simulink model "DriverInLoopSpeedgoat"  (R2021a)
settings: Solver=ode3  StartTime=0.0  StopTime=30  FixedStep=1e-3  RelTol=5e-3  EnableMultiTasking=on
StartFcn:
  | % tic
  | % tg2.start;
StopFcn:
  | % tg2.stop;
  | % toc
model workspace (MAT data in the model file):
  A_mu = 10
  B_reff = 8.386
  Cz = 7766.25
  DCT_Param : object (value not decoded)
  DLC_XEnd = 236.9
  DLC_XStart = 175.9
  DLC_YStart = 3.2153
  D_reff = 0.25826
  Downshift_Speeds = [9.5625 12.9375 16.3125 19.6875 23.0625 26.4375 29.8125 33.1875 36.5625 39.9375 43.3125 46.6875 ... (16 elements, 4x4)]
  EngRevLim = 7000
  Pedal_Positions = [0.1 0.4 0.5 0.9]
  SUS : object (value not decoded)
  Upshift_Speeds = [12.9375 16.3125 19.6875 33 26.4375 29.8125 33.1875 52.5 39.9375 43.3125 46.6875 77.25 ... (16 elements, 4x4)]
  VEH : object (value not decoded)
  V_o = 16.7
  V_xlow = 1
  WH : object (value not decoded)
  a = 1.4
  alpha_max = 1.5
  alpha_min = -1.5
  b = 1.8
  c_zo = 209651
  epsilon = 0.1
  h = 0.134
  path : object (value not decoded)
  pio = 220000
  q_Fcx = 0
  q_Fz2 = 15.4
  q_Fzy = 0
  q_reo = 0.9974
  q_sx1 = -0.007764
  q_sx10 = 0.2824
  q_sx11 = 5.349
  q_sx12 = 0
  q_sx13 = 0
  q_sx14 = 0
  q_sx2 = 1.1915
  q_sx3 = 0.013948
  q_sx4 = 4.912
  q_sx5 = 1.02
  q_sx6 = 22.83
  q_sx7 = 0.7104
  q_sx8 = -0.023393
  q_sx9 = 0.6581
  q_sy1 = 0.00702
  q_sy2 = 0
  q_sy3 = 0.001515
  q_sy4 = 8.514e-05
  q_sy5 = 0
  q_sy6 = 0
  q_sy7 = 0.9008
  q_sy8 = -0.4089
  q_v1 = 0.0007742
  q_v2 = 0.04667
  r_Bx1 = 12.531
  r_Bx2 = 9.532
  r_Bx3 = 0
  r_By1 = 10.615
  r_By2 = 7.705
  r_By3 = 3.433e-06
  r_By4 = 0
  r_Cx1 = 1.019
  r_Cy1 = 1.0585
  r_Ex1 = -0.4487
  r_Ex2 = -0.4726
  r_Ey1 = 0.3132
  r_Ey2 = 7.63e-06
  r_Hx1 = 0.0002374
  r_Hy1 = 0.011646
  r_Hy2 = 7.63e-06
  r_Vy1 = 0.05654
  r_Vy2 = 7.63e-06
  r_Vy3 = 0
  r_Vy4 = 99.9
  r_Vy5 = 2
  r_Vy6 = 15.814
  r_o = 0.3135
  vehWidth = 2
  w = 1
  xdot_ref = 13.4112
values from neighbouring files (symbols this model uses):
  stop_pedal = 20    [config_test.m]
symbols that are objects in the model workspace (value not decoded): VEH
undefined symbols (not defined in the file or in its folder): ESP_mode
libraries: autolibutils x7, simulink x6, slrealtimeutilitieslib x2, slrealtimeiplib x2, sim3dlib x1, sim3dautolib x1, pid_lib x1, slrealtimeobsoletelib x1, dspstat3 x1
(part 2 of 2)

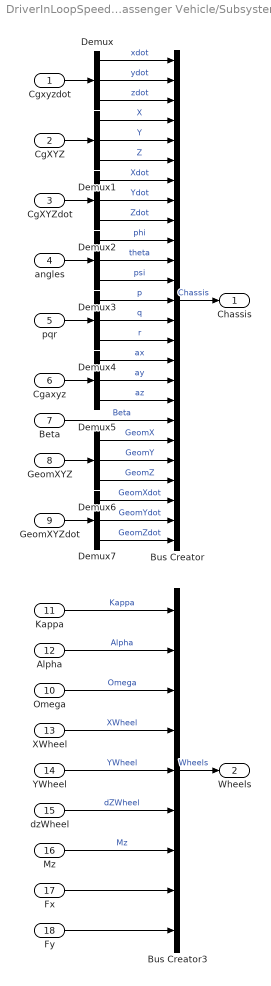
== system DriverInLoopSpeedgoat/Passenger Vehicle/Subsystem4 ==
  Cgxyzdot : Inport
  CgXYZ : Inport  Port=2
  CgXYZdot : Inport  Port=3
  angles : Inport  Port=4
  pqr : Inport  Port=5
  Cgaxyz : Inport  Port=6
  Beta : Inport  Port=7
  GeomXYZ : Inport  Port=8
  GeomXYZdot : Inport  Port=9
  Omega : Inport  Port=10
  Kappa : Inport  Port=11
  Alpha : Inport  Port=12
  XWheel : Inport  Port=13
  YWheel : Inport  Port=14
  dzWheel : Inport  Port=15
  Mz : Inport  Port=16
  Fx : Inport  Port=17
  Fy : Inport  Port=18
  Bus Creator : BusCreator  Inputs=25
  Bus Creator3 : BusCreator  Inputs=9
  Demux{,1..7} (8 alike) : Demux  Outputs=3
  Chassis : Outport  VectorParamsAs1DForOutWhenUnconnected=off
  Wheels : Outport  Port=2  VectorParamsAs1DForOutWhenUnconnected=off
  wires:
  Bus Creator/1 -> Chassis/1  "Chassis"
  Omega/1 -> Bus Creator3/3  "Omega"
  dzWheel/1 -> Bus Creator3/6  "dZWheel"
  Kappa/1 -> Bus Creator3/1  "Kappa"
  Bus Creator3/1 -> Wheels/1  "Wheels"
  YWheel/1 -> Bus Creator3/5  "YWheel"
  XWheel/1 -> Bus Creator3/4  "XWheel"
  Alpha/1 -> Bus Creator3/2  "Alpha"
  Cgxyzdot/1 -> Demux/1
  CgXYZ/1 -> Demux1/1
  CgXYZdot/1 -> Demux2/1
  angles/1 -> Demux3/1
  pqr/1 -> Demux4/1
  Cgaxyz/1 -> Demux5/1
  GeomXYZdot/1 -> Demux7/1
  GeomXYZ/1 -> Demux6/1
  Demux/1 -> Bus Creator/1  "xdot"
  Demux/2 -> Bus Creator/2  "ydot"
  Demux/3 -> Bus Creator/3  "zdot"
  Demux1/1 -> Bus Creator/4  "X"
  Demux1/2 -> Bus Creator/5  "Y"
  Demux1/3 -> Bus Creator/6  "Z"
  Demux2/1 -> Bus Creator/7  "Xdot"
  Demux2/2 -> Bus Creator/8  "Ydot"
  Demux2/3 -> Bus Creator/9  "Zdot"
  Demux3/1 -> Bus Creator/10  "phi"
  Demux3/2 -> Bus Creator/11  "theta"
  Demux3/3 -> Bus Creator/12  "psi"
  Demux4/1 -> Bus Creator/13  "p"
  Demux4/2 -> Bus Creator/14  "q"
  Demux4/3 -> Bus Creator/15  "r"
  Demux5/1 -> Bus Creator/16  "ax"
  Demux5/2 -> Bus Creator/17  "ay"
  Demux5/3 -> Bus Creator/18  "az"
  Beta/1 -> Bus Creator/19  "Beta"
  Demux6/1 -> Bus Creator/20  "GeomX"
  Demux6/2 -> Bus Creator/21  "GeomY"
  Demux6/3 -> Bus Creator/22  "GeomZ"
  Demux7/1 -> Bus Creator/23  "GeomXdot"
  Demux7/2 -> Bus Creator/24  "GeomYdot"
  Demux7/3 -> Bus Creator/25  "GeomZdot"
  Mz/1 -> Bus Creator3/7  "Mz"
  Fx/1 -> Bus Creator3/8
  Fy/1 -> Bus Creator3/9

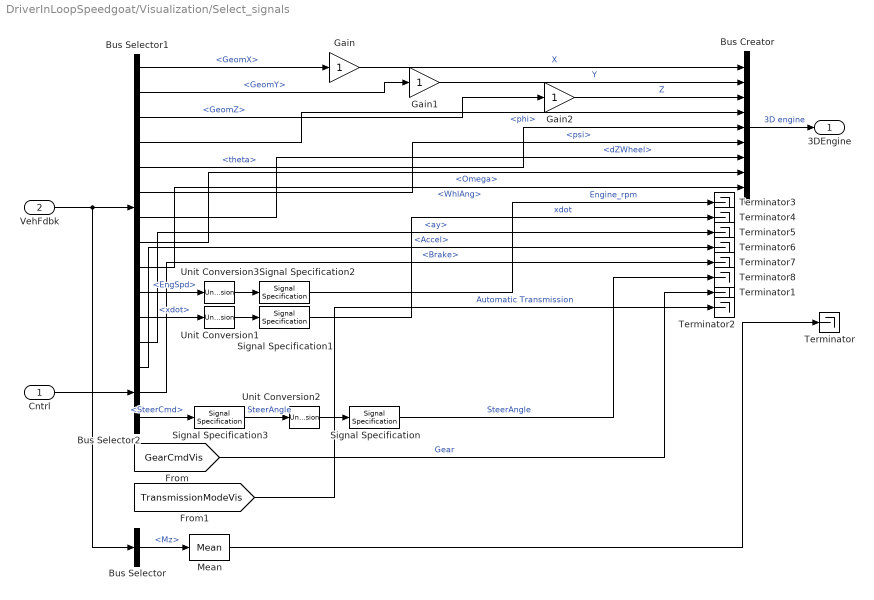
== system DriverInLoopSpeedgoat/Visualization/Select_signals ==
  Cntrl : Inport
  VehFdbk : Inport  Port=2
  Bus Creator : BusCreator  Inputs=9
  Bus Selector : BusSelector  OutputSignals=Wheels.Mz
  Bus Selector1 : BusSelector  OutputSignals=Body.GeomX,Body.GeomY,Body.GeomZ,Body.phi,Body.theta,Body.psi,Wheels.dZWheel,Wheels.Omega,Driveline.WhlAng,Driveline.EngSpd,Body.xdot,Body.ay
  Bus Selector2 : BusSelector  OutputSignals=Accel,Brake,SteerCmd
  Gain : Gain
  Gain1 : Gain
  Gain2 : Gain
  Mean : dspstat3/Mean  run=off  InputProcessing=Columns as channels (frame based)  reset_popup=None  directionMode=Each column  dimension=1  roiEnable=off  roiType=Rectangles  roiPortion=Entire ROI  roiOutput=Individual statistics for each ROI  roiFlag=off  roundingMode=Floor  overflowMode=off  outputDataTypeStr=Inherit: Same as accumulator  outputMin=[]  outputMax=[]  outputLastDataTypeStr=Inherit: Same as accumulator
  Signal Specification : SignalSpecification  Unit=deg
  Signal Specification1 : SignalSpecification  Unit=mph
  Signal Specification2 : SignalSpecification  Unit=rpm
  Signal Specification3 : SignalSpecification  Unit=deg
  Terminator{,1..8} (9 alike) : Terminator
  Unit Conversion1 : UnitConversion
  Unit Conversion2 : UnitConversion
  Unit Conversion3 : UnitConversion
  3DEngine : Outport
  wires:
  Bus Selector1/11 -> Unit Conversion1/1  "<xdot>"
  Signal Specification2/1 -> Terminator3/1  "Engine_rpm"
  Unit Conversion3/1 -> Signal Specification2/1
  Bus Selector2/1 -> Terminator6/1  "<Accel>"
  Bus Selector1/12 -> Terminator5/1  "<ay>"
  VehFdbk/1 -> Bus Selector1/1, Bus Selector/1
  Unit Conversion2/1 -> Signal Specification/1
  Signal Specification/1 -> Terminator8/1  "SteerAngle"
  Bus Selector1/8 -> Bus Creator/8  "<Omega>"
  Bus Selector1/4 -> Bus Creator/4  "<phi>"
  Cntrl/1 -> Bus Selector2/1
  Bus Selector1/10 -> Unit Conversion3/1  "<EngSpd>"
  Unit Conversion1/1 -> Signal Specification1/1
  Bus Selector2/3 -> Signal Specification3/1  "<SteerCmd>"
  Bus Selector1/5 -> Bus Creator/5  "<theta>"
  Bus Selector1/7 -> Bus Creator/7  "<dZWheel>"
  Bus Selector2/2 -> Terminator7/1  "<Brake>"
  Bus Selector1/6 -> Bus Creator/6  "<psi>"
  Bus Selector1/9 -> Bus Creator/9  "<WhlAng>"
  Signal Specification1/1 -> Terminator4/1  "xdot"
  Bus Selector/1 -> Mean/1  "<Mz>"
  Signal Specification3/1 -> Unit Conversion2/1  "SteerAngle"
  Bus Creator/1 -> 3DEngine/1  "3D engine"
  Mean/1 -> Terminator/1
  Bus Selector1/3 -> Gain2/1  "<GeomZ>"
  Bus Selector1/2 -> Gain1/1  "<GeomY>"
  [GearCmdVis] -> Terminator1/1  "Gear"
  Bus Selector1/1 -> Gain/1  "<GeomX>"
  [TransmissionModeVis] -> Terminator2/1  "Automatic Transmission"
  Gain/1 -> Bus Creator/1  "X"
  Gain1/1 -> Bus Creator/2  "Y"
  Gain2/1 -> Bus Creator/3  "Z"

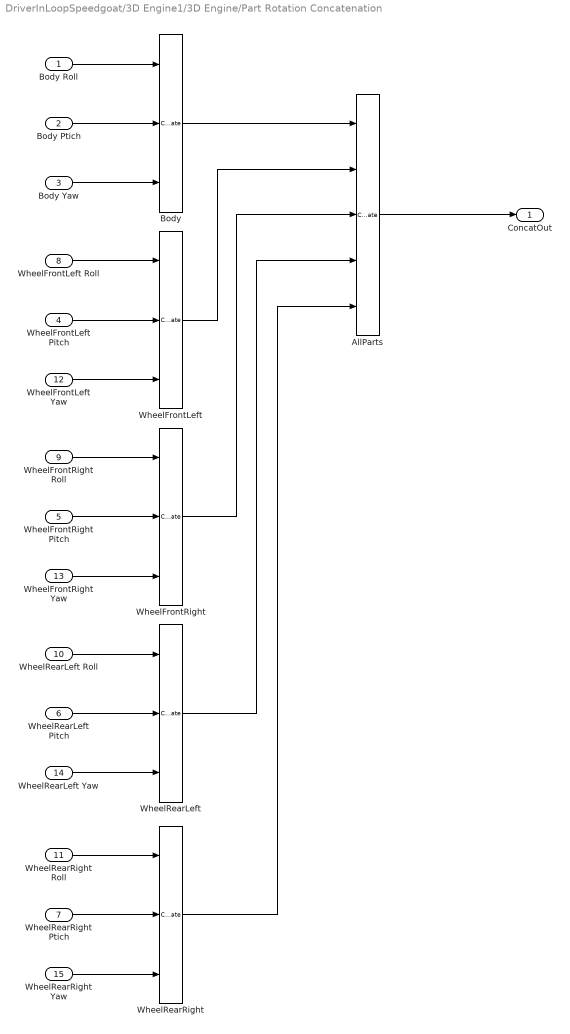
== system DriverInLoopSpeedgoat/3D Engine1/3D Engine/Part Rotation Concatenation ==
  Body Roll : Inport
  Body Ptich : Inport  Port=2
  Body Yaw : Inport  Port=3
  WheelFrontLeft Pitch : Inport  Port=4
  WheelFrontRight Pitch : Inport  Port=5
  WheelRearLeft Pitch : Inport  Port=6
  WheelRearRight Ptich : Inport  Port=7
  WheelFrontLeft Roll : Inport  Port=8
  WheelFrontRight Roll : Inport  Port=9
  WheelRearLeft Roll : Inport  Port=10
  WheelRearRight Roll : Inport  Port=11
  WheelFrontLeft Yaw : Inport  Port=12
  WheelFrontRight Yaw : Inport  Port=13
  WheelRearLeft Yaw : Inport  Port=14
  WheelRearRight Yaw : Inport  Port=15
  AllParts : Concatenate  NumInputs=5  Mode=Multidimensional array
  Body : Concatenate  NumInputs=3  Mode=Multidimensional array  ConcatenateDimension=2
  WheelFrontLeft : Concatenate  NumInputs=3  Mode=Multidimensional array  ConcatenateDimension=2
  WheelFrontRight : Concatenate  NumInputs=3  Mode=Multidimensional array  ConcatenateDimension=2
  WheelRearLeft : Concatenate  NumInputs=3  Mode=Multidimensional array  ConcatenateDimension=2
  WheelRearRight : Concatenate  NumInputs=3  Mode=Multidimensional array  ConcatenateDimension=2
  ConcatOut : Outport  VectorParamsAs1DForOutWhenUnconnected=off
  wires:
  Body Yaw/1 -> Body/3
  WheelFrontLeft Yaw/1 -> WheelFrontLeft/3
  WheelFrontLeft/1 -> AllParts/2
  Body/1 -> AllParts/1
  WheelRearLeft/1 -> AllParts/4
  WheelFrontRight/1 -> AllParts/3
  WheelRearRight Yaw/1 -> WheelRearRight/3
  WheelRearLeft Yaw/1 -> WheelRearLeft/3
  AllParts/1 -> ConcatOut/1
  WheelRearRight/1 -> AllParts/5
  WheelFrontRight Yaw/1 -> WheelFrontRight/3
  Body Roll/1 -> Body/1
  Body Ptich/1 -> Body/2
  WheelFrontLeft Pitch/1 -> WheelFrontLeft/2
  WheelFrontLeft Roll/1 -> WheelFrontLeft/1
  WheelFrontRight Roll/1 -> WheelFrontRight/1
  WheelFrontRight Pitch/1 -> WheelFrontRight/2
  WheelRearLeft Roll/1 -> WheelRearLeft/1
  WheelRearLeft Pitch/1 -> WheelRearLeft/2
  WheelRearRight Roll/1 -> WheelRearRight/1
  WheelRearRight Ptich/1 -> WheelRearRight/2

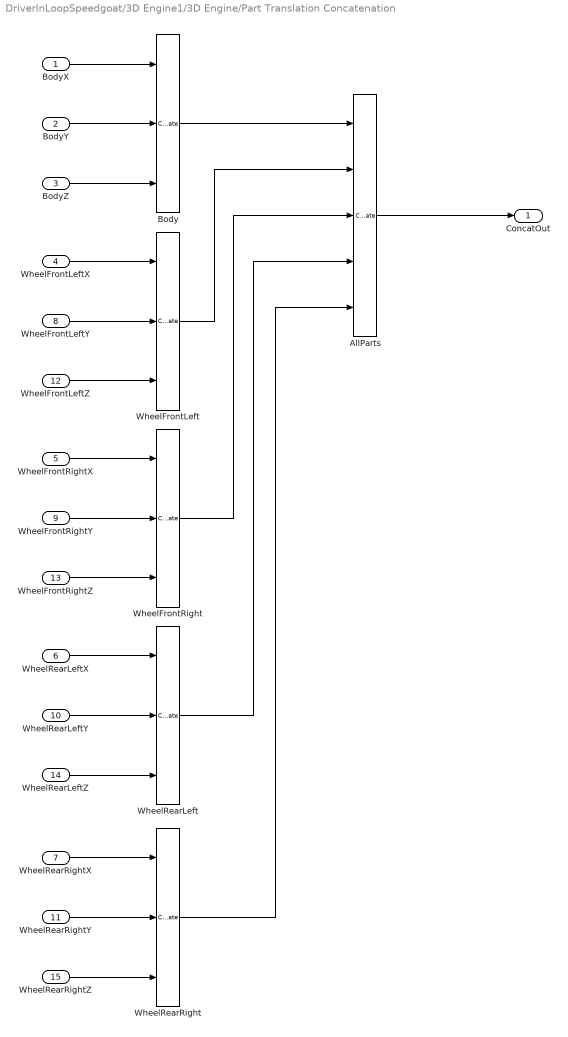
== system DriverInLoopSpeedgoat/3D Engine1/3D Engine/Part Translation Concatenation ==
  BodyX : Inport
  BodyY : Inport  Port=2
  BodyZ : Inport  Port=3
  WheelFrontLeftX : Inport  Port=4
  WheelFrontRightX : Inport  Port=5
  WheelRearLeftX : Inport  Port=6
  WheelRearRightX : Inport  Port=7
  WheelFrontLeftY : Inport  Port=8
  WheelFrontRightY : Inport  Port=9
  WheelRearLeftY : Inport  Port=10
  WheelRearRightY : Inport  Port=11
  WheelFrontLeftZ : Inport  Port=12
  WheelFrontRightZ : Inport  Port=13
  WheelRearLeftZ : Inport  Port=14
  WheelRearRightZ : Inport  Port=15
  AllParts : Concatenate  NumInputs=5  Mode=Multidimensional array
  Body : Concatenate  NumInputs=3  Mode=Multidimensional array  ConcatenateDimension=2
  WheelFrontLeft : Concatenate  NumInputs=3  Mode=Multidimensional array  ConcatenateDimension=2
  WheelFrontRight : Concatenate  NumInputs=3  Mode=Multidimensional array  ConcatenateDimension=2
  WheelRearLeft : Concatenate  NumInputs=3  Mode=Multidimensional array  ConcatenateDimension=2
  WheelRearRight : Concatenate  NumInputs=3  Mode=Multidimensional array  ConcatenateDimension=2
  ConcatOut : Outport  VectorParamsAs1DForOutWhenUnconnected=off
  wires:
  BodyX/1 -> Body/1
  BodyZ/1 -> Body/3
  WheelFrontLeftX/1 -> WheelFrontLeft/1
  WheelFrontLeftZ/1 -> WheelFrontLeft/3
  WheelFrontLeftY/1 -> WheelFrontLeft/2
  BodyY/1 -> Body/2
  WheelFrontLeft/1 -> AllParts/2
  WheelRearRightX/1 -> WheelRearRight/1
  Body/1 -> AllParts/1
  WheelRearLeft/1 -> AllParts/4
  WheelFrontRight/1 -> AllParts/3
  WheelRearRightZ/1 -> WheelRearRight/3
  WheelFrontRightY/1 -> WheelFrontRight/2
  WheelFrontRightX/1 -> WheelFrontRight/1
  WheelRearRightY/1 -> WheelRearRight/2
  WheelRearLeftZ/1 -> WheelRearLeft/3
  AllParts/1 -> ConcatOut/1
  WheelRearLeftY/1 -> WheelRearLeft/2
  WheelRearRight/1 -> AllParts/5
  WheelRearLeftX/1 -> WheelRearLeft/1
  WheelFrontRightZ/1 -> WheelFrontRight/3

== system DriverInLoopSpeedgoat/3D Engine1/3D Engine/Scale ==
  Constant{1..12,17,32..33} (15 alike) : Constant  OutDataTypeStr=single
  PartConcatenation : Subsystem
  ScaleOut : Outport  VectorParamsAs1DForOutWhenUnconnected=off
  wires:
  Constant10/1 -> PartConcatenation/15(WheelRearRightZ)
  Constant9/1 -> PartConcatenation/14(WheelRearRightY)
  Constant11/1 -> PartConcatenation/13(WheelRearRightX)
  Constant7/1 -> PartConcatenation/12(WheelRearLeftZ)
  Constant6/1 -> PartConcatenation/11(WheelRearLeftY)
  Constant8/1 -> PartConcatenation/10(WheelRearLeftX)
  Constant4/1 -> PartConcatenation/9(WheelFrontRightZ)
  Constant3/1 -> PartConcatenation/8(WheelFrontRightY)
  Constant5/1 -> PartConcatenation/7(WheelFrontRightX)
  Constant2/1 -> PartConcatenation/6(WheelFrontLeftZ)
  Constant1/1 -> PartConcatenation/5(WheelFrontLeftY)
  Constant33/1 -> PartConcatenation/4(WheelFrontLeftX)
  Constant32/1 -> PartConcatenation/3(BodyZ)
  Constant17/1 -> PartConcatenation/2(BodyY)
  Constant12/1 -> PartConcatenation/1(BodyX)
  PartConcatenation/1(ConcatOut) -> ScaleOut/1

== system DriverInLoopSpeedgoat/Controllers/Brake Controller/Bang Bang ABS ==
  Pref : Inport
  xdot : Inport  Port=2
  <Kappa> : Inport  Port=3
  Abs : Abs
  Add : Sum  Inputs=-+
  Bang-bang controller : Subsystem  mask(Sign){}
      mask help: y = sign(x)
      mask Help: Sign Function:\n\t\t\ty = 1 if x > 0\n\t\t\ty = 0 if x = 0\n\t\t\ty = -1 if x < 0
      mask Display: plot(-50,-50,50,50,[-50,50],[0,0],[0,0],[-50,50],[-40,0],[-30,-30],[0,40],[30,30])
  Compare To Constant : simulink/Logic and Bit Operations/Compare To Constant  relop=>=  const=.2  OutDataTypeStr=boolean
  Compare To Constant1 : simulink/Logic and Bit Operations/Compare To Constant  relop=>=  const=.75  OutDataTypeStr=boolean
  Compare To Constant2 : simulink/Logic and Bit Operations/Compare To Constant  relop=>=  const=.5  OutDataTypeStr=boolean
  Constant : Constant  Value=.25
  Debounce : autolibutils/Debounce  DbcOn_Cnts=.1*.001  DbcOff_Cnts=.1*.001  aMode=aMode
      settings: SourceProductBaseCode=PW,DR,MT,UV,VE
  Gain : Gain  Gain=200
  Logical Operator : Logic  Inputs=3  AllPortsSameDT=off  OutDataTypeStr=boolean
  Rate Transition : RateTransition  OutPortSampleTime=.001
  Rate Transition1 : RateTransition
  Switch : Switch  Criteria=u2 > Threshold  ZeroCross=off
  PCmd : Outport  VectorParamsAs1DForOutWhenUnconnected=off
  wires:
  Bang-bang controller/1(out_1) -> Gain/1
  Add/1 -> Bang-bang controller/1(in_1)
  Rate Transition1/1 -> PCmd/1
  <Kappa>/1 -> Rate Transition/1
  Pref/1 -> Switch/3, Compare To Constant1/1  "Pref"
  Constant/1 -> Add/2  "slip ref"
  Switch/1 -> Rate Transition1/1
  Rate Transition/1 -> Add/1, Compare To Constant/1
  Logical Operator/1 -> Debounce/1
  Compare To Constant/1 -> Logical Operator/2
  Compare To Constant1/1 -> Logical Operator/3
  Debounce/1 -> Switch/2
  xdot/1 -> Abs/1
  Abs/1 -> Compare To Constant2/1
  Compare To Constant2/1 -> Logical Operator/1
  Gain/1 -> Switch/1

== system DriverInLoopSpeedgoat/Controllers/ECU/Rev Limiter Control ==
  TrqCmd : Inport
  EngSpd : Inport  Port=2
  1-D Lookup Table : Lookup_n-D  NumberOfTableDimensions=1  BreakpointsForDimension1=[1 1.01]  Table=[1 0]  ExtrapMethod=Clip  InternalRulePriority=Speed  RndMeth=Simplest  InputSameDT=on
  Constant : Constant  Value=EngRevLim
  Product : Product
  Product1 : Product  Inputs=*/
  TrqCmdRevLimited : Outport  VectorParamsAs1DForOutWhenUnconnected=off
  wires:
  EngSpd/1 -> Product1/1
  Product/1 -> TrqCmdRevLimited/1
  1-D Lookup Table/1 -> Product/2
  TrqCmd/1 -> Product/1
  Constant/1 -> Product1/2
  Product1/1 -> 1-D Lookup Table/1

== system DriverInLoopSpeedgoat/Controllers/Transmission Controller/Automatic ==
  Accel : Inport
  EngSpd : Inport  Port=2  Unit=rad/s
  PrpSpd : Inport  Port=3
  Action Port : ActionPort  ActionPortLabel=case [ 1 ]:
  Neutral Select : Subsystem
  Prop Shaft Speed LPF : DiscreteTransferFcn  Numerator=[0.000000000000000 0.009950166250832 ]  Denominator=[1.000000000000000 -0.990049833749168 ]  mask(DiscretizedDiscreteTransferFcn){}
      mask init:
      | %zoh
  Signal Specification : SignalSpecification  Unit=rpm
  TCM Shift Controller : Stateflow chart  TreatAsAtomicUnit=on
  Unit Conversion : UnitConversion
  prop speed to vehicle speed : Gain  Gain=0.45
  Gear : Outport  VectorParamsAs1DForOutWhenUnconnected=off
  wires:
  TCM Shift Controller/1(GearCmd) -> Gear/1
  Unit Conversion/1 -> Signal Specification/1
  PrpSpd/1 -> Prop Shaft Speed LPF/1
  Signal Specification/1 -> Neutral Select/2(EngSpd)  "EngSpd"
  EngSpd/1 -> Unit Conversion/1
  Accel/1 -> Neutral Select/1(AccCmd), TCM Shift Controller/2(pedal)  "AccCmd"
  Prop Shaft Speed LPF/1 -> prop speed to vehicle speed/1
  prop speed to vehicle speed/1 -> TCM Shift Controller/1(speed)
  Neutral Select/1(Neutral Select) -> TCM Shift Controller/3(Neutral)

== system DriverInLoopSpeedgoat/Controllers/Transmission Controller/Paddles ==
  UpReq : Inport
  DownReq : Inport  Port=2  Unit=rad/s
  Action Port : ActionPort  ActionPortLabel=case [ 0 ]:
  Add1 : Sum  Inputs=+-+
  Current Gear : UnitDelay  SampleTime=-1  HasFrameUpgradeWarning=on
  Data Type Conversion2 : DataTypeConversion  OutDataTypeStr=int8
  Debounce : autolibutils/Debounce  DbcOn_Cnts=10  DbcOff_Cnts=10  aMode=aMode
      settings: SourceProductBaseCode=PW,DR,MT,UV,VE
  Debounce1 : autolibutils/Debounce  DbcOn_Cnts=10  DbcOff_Cnts=10  aMode=aMode
      settings: SourceProductBaseCode=PW,DR,MT,UV,VE
  Demux : Demux  Outputs=2
  Detect Increase2 : simulink/Logic and Bit Operations/Detect Increase  vinit=0.0  OutDataTypeStr=boolean
  Logical Operator1 : Logic  Operator=XOR  Inputs=1  AllPortsSameDT=off  OutDataTypeStr=boolean
  Mux : Mux  Inputs=2
  Saturation : Saturate  UpperLimit=5  LowerLimit=-1
  Switch2 : Switch  Criteria=u2 > Threshold
  Gear : Outport  VectorParamsAs1DForOutWhenUnconnected=off
  wires:
  Saturation/1 -> Gear/1, Current Gear/1
  UpReq/1 -> Debounce/1
  Current Gear/1 -> Add1/3, Switch2/3
  Debounce1/1 -> Mux/2
  Data Type Conversion2/1 -> Demux/1
  Add1/1 -> Switch2/1
  Mux/1 -> Detect Increase2/1
  Detect Increase2/1 -> Data Type Conversion2/1, Logical Operator1/1
  Logical Operator1/1 -> Switch2/2
  Debounce/1 -> Mux/1
  DownReq/1 -> Debounce1/1
  Demux/2 -> Add1/2
  Demux/1 -> Add1/1
  Switch2/1 -> Saturation/1

== system DriverInLoopSpeedgoat/Environment/Friction Scaling/Constant ==
  Bus Creator2 : BusCreator  Inputs=4
  Constant Mu : Constant  Value=ones(4,1).*1
  Demux1 : Demux
  Signal Specification1 : SignalSpecification  Unit=1
  mu : Outport  VectorParamsAs1DForOutWhenUnconnected=off
  wires:
  Demux1/3 -> Bus Creator2/3  "mu_RL"
  Demux1/4 -> Bus Creator2/4  "mu_RR"
  Demux1/1 -> Bus Creator2/1  "mu_FL"
  Demux1/2 -> Bus Creator2/2  "mu_FR"
  Bus Creator2/1 -> mu/1  "mu"
  Constant Mu/1 -> Signal Specification1/1
  Signal Specification1/1 -> Demux1/1

== system DriverInLoopSpeedgoat/Environment/Friction Scaling/Lookup Table ==
  VehFdbk : Inport
  Bus Creator2 : BusCreator  Inputs=4
  Bus Creator3 : BusCreator  Inputs=1
  Bus Selector : BusSelector  OutputSignals=Wheels.XWheel,Wheels.YWheel
  Demux1 : Demux
  Memory : Memory
  Memory1 : Memory
  Split Mu : Subsystem  TreatAsAtomicUnit=on
  mu : Outport  VectorParamsAs1DForOutWhenUnconnected=off
  wires:
  Demux1/1 -> Bus Creator2/1  "mu_FL"
  Demux1/3 -> Bus Creator2/3  "mu_RL"
  Demux1/4 -> Bus Creator2/4  "mu_RR"
  Demux1/2 -> Bus Creator2/2  "mu_FR"
  Bus Creator2/1 -> Bus Creator3/1  "mu"
  Bus Creator3/1 -> mu/1
  Memory/1 -> Split Mu/1(In1)
  Bus Selector/1 -> Memory/1  "<XWheel>"
  Memory1/1 -> Split Mu/2(In2)
  Bus Selector/2 -> Memory1/1  "<YWheel>"
  VehFdbk/1 -> Bus Selector/1
  Split Mu/1(Out1) -> Demux1/1

== system DriverInLoopSpeedgoat/Environment/Ground Height/3D Engine ==
  Bus Creator : BusCreator  Inputs=4
  Data Type Conversion : DataTypeConversion
  Data Type Conversion1 : DataTypeConversion  OutDataTypeStr=boolean
  Demux : Demux
  Signal Specification : SignalSpecification  Unit=m
  Subsystem : Subsystem
  While Iterator Subsystem : Subsystem  TreatAsAtomicUnit=on
  z : Outport  VectorParamsAs1DForOutWhenUnconnected=off
  wires:
  Demux/2 -> Bus Creator/2  "G_FR_z"
  Demux/1 -> Bus Creator/1  "G_FL_z"
  Demux/4 -> Bus Creator/4  "G_RR_z"
  Demux/3 -> Bus Creator/3  "G_RL_z"
  Bus Creator/1 -> z/1  "z"
  Data Type Conversion/1 -> Signal Specification/1
  Signal Specification/1 -> Demux/1
  Subsystem/1(Rx Data) -> Data Type Conversion/1
  While Iterator Subsystem/1(Data) -> Subsystem/1(In1)
  Data Type Conversion1/1 -> Subsystem/Enable
  While Iterator Subsystem/2(NumMsg) -> Data Type Conversion1/1

== system DriverInLoopSpeedgoat/Environment/Ground Height/Constant ==
  Bus Creator : BusCreator  Inputs=4
  Bus Creator3 : BusCreator  Inputs=1
  Constant1 : Constant  Value=zeros(4,1)
  Demux : Demux
  Signal Specification : SignalSpecification  Unit=m
  z : Outport  VectorParamsAs1DForOutWhenUnconnected=off
  wires:
  Constant1/1 -> Signal Specification/1
  Signal Specification/1 -> Demux/1
  Demux/4 -> Bus Creator/4  "G_RR_z"
  Demux/1 -> Bus Creator/1  "G_FL_z"
  Demux/3 -> Bus Creator/3  "G_RL_z"
  Demux/2 -> Bus Creator/2  "G_FR_z"
  Bus Creator/1 -> Bus Creator3/1  "z"
  Bus Creator3/1 -> z/1

== system DriverInLoopSpeedgoat/External Driver Input/External Driver - Host/Receive UDP ==
  Compare To Constant : simulink/Logic and Bit Operations/Compare To Constant  relop===  const=19  OutDataTypeStr=boolean
  Constant : Constant  OutDataTypeStr=Inherit: Inherit via back propagation  SampleTime=-1
  Receive : slrealtimeiplib/UDP Receive  useHostTargetConn=on  ipAddress=target_ip  localPort=25003  rcvWidth=19  rcvFmAny=off  fmAddress=host_ip  sampleTime=-1
      settings: SourceProductBaseCode=XP
  Subtract : Sum  Inputs=+-
  While Iterator : WhileIterator  MaxIters=10  WhileBlockType=do-while  ShowIterationPort=on
  NumMsg : Outport
  Data : Outport  Port=2
  wires:
  Receive/2 -> Compare To Constant/1
  Compare To Constant/1 -> While Iterator/1
  While Iterator/1 -> Subtract/1
  Constant/1 -> Subtract/2
  Receive/1 -> Data/1
  Subtract/1 -> NumMsg/1

== system DriverInLoopSpeedgoat/External Driver Input/External Driver - Host/Subsystem ==
  In1 : Inport
  Enable : EnablePort
  Byte Unpacking : slrealtimeutilitieslib/Byte Unpacking  MaskUnpackedDataTypes={'double','double','boolean','boolean','boolean'}  MaskUnpackedDataSizes={[1],[1],[1],[1],[1]}  MaskAlignment=1
      settings: SourceProductBaseCode=XP
  Steer : Outport
  AccelBrake : Outport  Port=2
  ShiftDn : Outport  Port=3
  ShiftUp : Outport  Port=4
  ToggleMode : Outport  Port=5
  wires:
  In1/1 -> Byte Unpacking/1
  Byte Unpacking/2 -> AccelBrake/1  "AccelBrake"
  Byte Unpacking/3 -> ShiftDn/1  "ShiftDn"
  Byte Unpacking/4 -> ShiftUp/1  "ShiftUp"
  Byte Unpacking/1 -> Steer/1  "Steer"
  Byte Unpacking/5 -> ToggleMode/1  "Toggle"

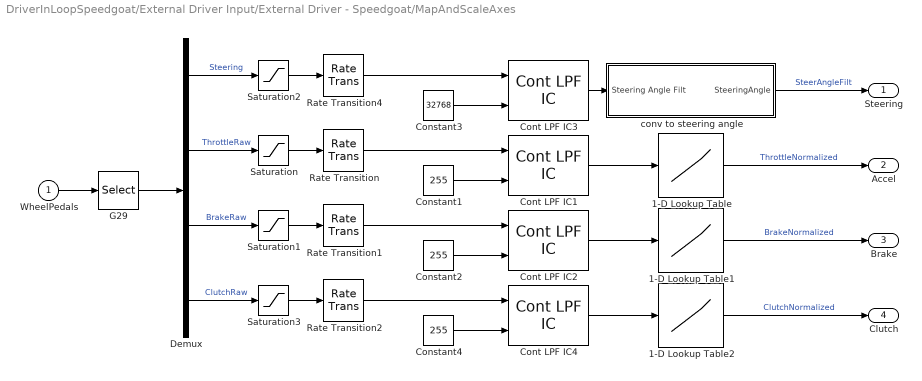
== system DriverInLoopSpeedgoat/External Driver Input/External Driver - Speedgoat/MapAndScaleAxes ==
  WheelPedals : Inport
  1-D Lookup Table : Lookup_n-D  NumberOfTableDimensions=1  BreakpointsForDimension1=[0 255]  Table=[1 0]  ExtrapMethod=Clip  UseLastTableValue=on  InternalRulePriority=Speed  RndMeth=Simplest  InputSameDT=on
  1-D Lookup Table1 : Lookup_n-D  NumberOfTableDimensions=1  BreakpointsForDimension1=[0 255]  Table=[1 0]  ExtrapMethod=Clip  UseLastTableValue=on  InternalRulePriority=Speed  RndMeth=Simplest  InputSameDT=on
  1-D Lookup Table2 : Lookup_n-D  NumberOfTableDimensions=1  BreakpointsForDimension1=[0 255]  Table=[1 0]  ExtrapMethod=Clip  UseLastTableValue=on  InternalRulePriority=Speed  RndMeth=Simplest  InputSameDT=on
  Constant1 : Constant  Value=255
  Constant2 : Constant  Value=255
  Constant3 : Constant  Value=32768
  Constant4 : Constant  Value=255
  Cont LPF IC1 : autolibutils/Cont LPF IC  wc=8*pi  aMode=aMode  dataType=off
      settings: SourceProductBaseCode=PW,DR,MT,UV,VE
  Cont LPF IC2 : autolibutils/Cont LPF IC  wc=8*pi  aMode=aMode  dataType=off
      settings: SourceProductBaseCode=PW,DR,MT,UV,VE
  Cont LPF IC3 : autolibutils/Cont LPF IC  wc=10  aMode=aMode  dataType=off
      settings: SourceProductBaseCode=PW,DR,MT,UV,VE
  Cont LPF IC4 : autolibutils/Cont LPF IC  wc=8*pi  aMode=aMode  dataType=off
      settings: SourceProductBaseCode=PW,DR,MT,UV,VE
  Demux : Demux
  G29 : Selector  InputPortWidth=4  IndexOptions=Index vector (dialog)  Indices=[1 2 3 4]  OutputSizes=1
  Rate Transition : RateTransition  Integrity=off  InitialCondition=4095
  Rate Transition1 : RateTransition  Integrity=off  InitialCondition=4095
  Rate Transition2 : RateTransition  Integrity=off  InitialCondition=4095
  Rate Transition4 : RateTransition  Integrity=off  Deterministic=off  InitialCondition=4095
  Saturation : Saturate  UpperLimit=255  LowerLimit=0
  Saturation1 : Saturate  UpperLimit=255  LowerLimit=0
  Saturation2 : Saturate  UpperLimit=65535  LowerLimit=0
  Saturation3 : Saturate  UpperLimit=4096  LowerLimit=0
  conv to steering angle : Subsystem
  Steering : Outport  VectorParamsAs1DForOutWhenUnconnected=off
  Accel : Outport  Port=2  VectorParamsAs1DForOutWhenUnconnected=off
  Brake : Outport  Port=3  VectorParamsAs1DForOutWhenUnconnected=off
  Clutch : Outport  Port=4  VectorParamsAs1DForOutWhenUnconnected=off
  wires:
  WheelPedals/1 -> G29/1
  1-D Lookup Table2/1 -> Clutch/1  "ClutchNormalized"
  conv to steering angle/1(SteeringAngle) -> Steering/1  "SteerAngleFilt"
  Constant2/1 -> Cont LPF IC2/2
  Constant3/1 -> Cont LPF IC3/2
  Demux/2 -> Saturation/1  "ThrottleRaw"
  Demux/1 -> Saturation2/1  "Steering"
  Cont LPF IC2/1 -> 1-D Lookup Table1/1
  Demux/4 -> Saturation3/1  "ClutchRaw"
  1-D Lookup Table/1 -> Accel/1  "ThrottleNormalized"
  Cont LPF IC1/1 -> 1-D Lookup Table/1
  Cont LPF IC4/1 -> 1-D Lookup Table2/1
  Demux/3 -> Saturation1/1  "BrakeRaw"
  1-D Lookup Table1/1 -> Brake/1  "BrakeNormalized"
  Constant1/1 -> Cont LPF IC1/2
  Constant4/1 -> Cont LPF IC4/2
  G29/1 -> Demux/1
  Saturation3/1 -> Rate Transition2/1
  Saturation1/1 -> Rate Transition1/1
  Saturation/1 -> Rate Transition/1
  Saturation2/1 -> Rate Transition4/1
  Rate Transition/1 -> Cont LPF IC1/1
  Rate Transition1/1 -> Cont LPF IC2/1
  Rate Transition2/1 -> Cont LPF IC4/1
  Rate Transition4/1 -> Cont LPF IC3/1
  Cont LPF IC3/1 -> conv to steering angle/1(Steering Angle Filt)

== system DriverInLoopSpeedgoat/External Driver Input/External Driver - Speedgoat/MapButtons ==
  Buttons : Inport
  Data Type Conversion : DataTypeConversion
  Data Type Conversion1 : DataTypeConversion
  Demux3 : Demux  Outputs=2
  G29 : Selector  InputPortWidth=13  IndexOptions=Index vector (dialog)  Indices=[5 6 1 2 3 4 7 8 9 10 11 12 13]  OutputSizes=1
  Select Left and Right Shift Paddle buttons : Selector  InputPortWidth=13  IndexOptions=Index vector (dialog)  Indices=[1 2]  OutputSizes=1
  LeftPaddle : Outport  VectorParamsAs1DForOutWhenUnconnected=off
  RightPaddle : Outport  Port=2  VectorParamsAs1DForOutWhenUnconnected=off
  AllButtons : Outport  Port=3  VectorParamsAs1DForOutWhenUnconnected=off
  wires:
  Buttons/1 -> G29/1
  Data Type Conversion/1 -> LeftPaddle/1
  Data Type Conversion1/1 -> RightPaddle/1
  Demux3/1 -> Data Type Conversion/1  "Left Paddle"
  Demux3/2 -> Data Type Conversion1/1  "Right Paddle"
  Select Left and Right Shift Paddle buttons/1 -> Demux3/1
  G29/1 -> AllButtons/1, Select Left and Right Shift Paddle buttons/1

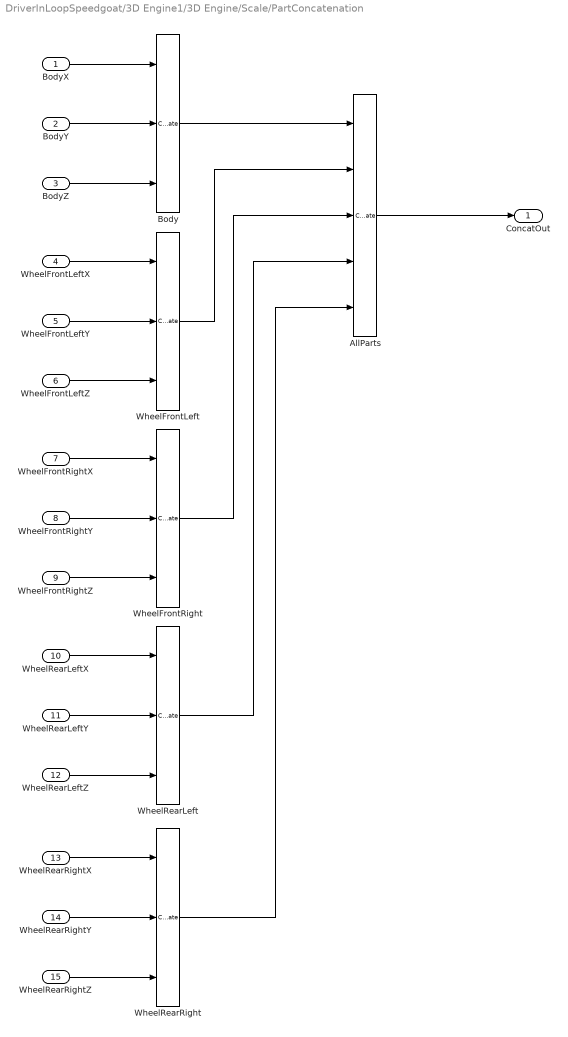
== system DriverInLoopSpeedgoat/3D Engine1/3D Engine/Scale/PartConcatenation ==
  BodyX : Inport
  BodyY : Inport  Port=2
  BodyZ : Inport  Port=3
  WheelFrontLeftX : Inport  Port=4
  WheelFrontLeftY : Inport  Port=5
  WheelFrontLeftZ : Inport  Port=6
  WheelFrontRightX : Inport  Port=7
  WheelFrontRightY : Inport  Port=8
  WheelFrontRightZ : Inport  Port=9
  WheelRearLeftX : Inport  Port=10
  WheelRearLeftY : Inport  Port=11
  WheelRearLeftZ : Inport  Port=12
  WheelRearRightX : Inport  Port=13
  WheelRearRightY : Inport  Port=14
  WheelRearRightZ : Inport  Port=15
  AllParts : Concatenate  NumInputs=5  Mode=Multidimensional array
  Body : Concatenate  NumInputs=3  Mode=Multidimensional array  ConcatenateDimension=2
  WheelFrontLeft : Concatenate  NumInputs=3  Mode=Multidimensional array  ConcatenateDimension=2
  WheelFrontRight : Concatenate  NumInputs=3  Mode=Multidimensional array  ConcatenateDimension=2
  WheelRearLeft : Concatenate  NumInputs=3  Mode=Multidimensional array  ConcatenateDimension=2
  WheelRearRight : Concatenate  NumInputs=3  Mode=Multidimensional array  ConcatenateDimension=2
  ConcatOut : Outport  VectorParamsAs1DForOutWhenUnconnected=off
  wires:
  BodyX/1 -> Body/1
  BodyZ/1 -> Body/3
  WheelFrontLeftX/1 -> WheelFrontLeft/1
  WheelFrontLeftZ/1 -> WheelFrontLeft/3
  WheelFrontLeftY/1 -> WheelFrontLeft/2
  BodyY/1 -> Body/2
  WheelFrontLeft/1 -> AllParts/2
  WheelRearRightX/1 -> WheelRearRight/1
  Body/1 -> AllParts/1
  WheelRearLeft/1 -> AllParts/4
  WheelFrontRight/1 -> AllParts/3
  WheelRearRightZ/1 -> WheelRearRight/3
  WheelFrontRightY/1 -> WheelFrontRight/2
  WheelFrontRightX/1 -> WheelFrontRight/1
  WheelRearRightY/1 -> WheelRearRight/2
  WheelRearLeftZ/1 -> WheelRearLeft/3
  AllParts/1 -> ConcatOut/1
  WheelRearLeftY/1 -> WheelRearLeft/2
  WheelRearRight/1 -> AllParts/5
  WheelRearLeftX/1 -> WheelRearLeft/1
  WheelFrontRightZ/1 -> WheelFrontRight/3

== system DriverInLoopSpeedgoat/Controllers/Brake Controller/Bang Bang ABS/Bang-bang controller ==
  in_1 : Inport
  Constant : Constant  Value=0
  Data Type Conversion1 : DataTypeConversion  OutDataTypeStr=double  SaturateOnIntegerOverflow=on  RndMeth=Zero
  Data Type Conversion2 : DataTypeConversion  OutDataTypeStr=double  SaturateOnIntegerOverflow=on  RndMeth=Zero
  Relational Operator : RelationalOperator  Operator=>  OutDataTypeStr=boolean  RndMeth=Nearest  InputSameDT=on
  Relational Operator1 : RelationalOperator  Operator=<  OutDataTypeStr=boolean  RndMeth=Nearest  InputSameDT=on
  Sum : Sum  Inputs=+-  InputSameDT=on  SaturateOnIntegerOverflow=on  OutDataTypeStr=Inherit: Same as first input
  out_1 : Outport  VectorParamsAs1DForOutWhenUnconnected=off
  wires:
  Data Type Conversion2/1 -> Sum/2
  Data Type Conversion1/1 -> Sum/1
  Sum/1 -> out_1/1
  Relational Operator/1 -> Data Type Conversion1/1
  Relational Operator1/1 -> Data Type Conversion2/1
  Constant/1 -> Relational Operator/2, Relational Operator1/2
  in_1/1 -> Relational Operator1/1, Relational Operator/1

== system DriverInLoopSpeedgoat/Controllers/Transmission Controller/Automatic/Neutral Select ==
  AccCmd : Inport
  EngSpd : Inport  Port=2
  Constant : Constant  Value=1200
  Constant1 : Constant  Value=1e-6
  Logical Operator : Logic  AllPortsSameDT=off  OutDataTypeStr=boolean
  Relational Operator : RelationalOperator  Operator=<=  OutDataTypeStr=boolean  RndMeth=Simplest
  Relational Operator1 : RelationalOperator  Operator=<=  OutDataTypeStr=boolean  RndMeth=Simplest
  Neutral Select : Outport  VectorParamsAs1DForOutWhenUnconnected=off
  wires:
  EngSpd/1 -> Relational Operator/1
  Relational Operator1/1 -> Logical Operator/1
  AccCmd/1 -> Relational Operator1/1
  Constant1/1 -> Relational Operator1/2
  Logical Operator/1 -> Neutral Select/1
  Constant/1 -> Relational Operator/2
  Relational Operator/1 -> Logical Operator/2

== system DriverInLoopSpeedgoat/Controllers/Transmission Controller/Automatic/TCM Shift Controller/calc ==
  note: Determine if next gear will be
      | higher or lower than current gear
  gear : Inport
  pedal : Inport  Port=2
  speed : Inport  Port=3
  f : TriggerPort  TriggerType=function-call  VariantControl=Variant  StatesWhenEnabling=reset
      settings: CopyFcn=Stateflow.SLINSF.SimulinkMan.removeBlockPreDeleteFcn  PreDeleteFcn=Stateflow.SLINSF.SimulinkMan.unsafePredeleteFcn
  Add1 : Sum  Inputs=+-
  Add3 : Sum  Inputs=+-
  Add4 : Sum  Inputs=+-
  Calculate Upshift Threshold : Lookup_n-D  BreakpointsForDimension1=Pedal_Positions  BreakpointsForDimension2=1:4  Table=Upshift_Speeds  ExtrapMethod=Clip  UseLastTableValue=on  InternalRulePriority=Speed  RndMeth=Simplest  InputSameDT=on
      settings: InputPortMap=u0,u1
  Calculate Downshift Threshold : Lookup_n-D  BreakpointsForDimension1=Pedal_Positions  BreakpointsForDimension2=2:5  Table=Downshift_Speeds  ExtrapMethod=Clip  UseLastTableValue=on  InternalRulePriority=Speed  RndMeth=Simplest  InputSameDT=on
      settings: InputPortMap=u0,u1
  SpdThr : Outport  VectorParamsAs1DForOutWhenUnconnected=off
  wires:
  pedal/1 -> Calculate Downshift Threshold/1, Calculate Upshift Threshold/1
  gear/1 -> Calculate Downshift Threshold/2, Calculate Upshift Threshold/2
  Calculate Downshift Threshold/1 -> Add3/2
  Calculate Upshift Threshold/1 -> Add1/1
  speed/1 -> Add1/2, Add3/1
  Add1/1 -> Add4/1
  Add3/1 -> Add4/2
  Add4/1 -> SpdThr/1

== system DriverInLoopSpeedgoat/Controllers/Transmission Controller/Automatic/TCM Shift Controller/calc_down ==
  gear : Inport
  pedal : Inport  Port=2
  f : TriggerPort  TriggerType=function-call  VariantControl=Variant  StatesWhenEnabling=reset
      settings: CopyFcn=Stateflow.SLINSF.SimulinkMan.removeBlockPreDeleteFcn  PreDeleteFcn=Stateflow.SLINSF.SimulinkMan.unsafePredeleteFcn
  Calculate Downshift Threshold : Lookup_n-D  BreakpointsForDimension1=Pedal_Positions  BreakpointsForDimension2=2:5  Table=Downshift_Speeds  ExtrapMethod=Clip  UseLastTableValue=on  InternalRulePriority=Speed  RndMeth=Simplest  InputSameDT=on
      settings: InputPortMap=u0,u1
  down_th : Outport  VectorParamsAs1DForOutWhenUnconnected=off
  wires:
  Calculate Downshift Threshold/1 -> down_th/1
  gear/1 -> Calculate Downshift Threshold/2
  pedal/1 -> Calculate Downshift Threshold/1

== system DriverInLoopSpeedgoat/Controllers/Transmission Controller/Automatic/TCM Shift Controller/calc_up ==
  gear : Inport
  pedal : Inport  Port=2
  f : TriggerPort  TriggerType=function-call  VariantControl=Variant  StatesWhenEnabling=reset
      settings: CopyFcn=Stateflow.SLINSF.SimulinkMan.removeBlockPreDeleteFcn  PreDeleteFcn=Stateflow.SLINSF.SimulinkMan.unsafePredeleteFcn
  Calculate Upshift Threshold : Lookup_n-D  BreakpointsForDimension1=Pedal_Positions  BreakpointsForDimension2=1:4  Table=Upshift_Speeds  ExtrapMethod=Clip  UseLastTableValue=on  InternalRulePriority=Speed  RndMeth=Simplest  InputSameDT=on
      settings: InputPortMap=u0,u1
  up_th : Outport  VectorParamsAs1DForOutWhenUnconnected=off
  wires:
  Calculate Upshift Threshold/1 -> up_th/1
  pedal/1 -> Calculate Upshift Threshold/1
  gear/1 -> Calculate Upshift Threshold/2

== system DriverInLoopSpeedgoat/Environment/Friction Scaling/Lookup Table/Split Mu ==
  In1 : Inport  Partition=on  PartitionDimension=1  PartitionWidth=1  PartitionOffset=0
  In2 : Inport  Port=2  Partition=on  PartitionDimension=1  PartitionWidth=1  PartitionOffset=0
  2-D Lookup Table : Lookup_n-D  BreakpointsForDimension1=[0,50,51,1000]  BreakpointsForDimension2=[-5,0,0.1,5]+VEH.InitialLatPosition  Table=reshape([1,1,0.6,0.6,1,1,0.6,0.6,1,1,1,1,1,1,1,1],4,4).*1.1  InternalRulePriority=Speed  RndMeth=Simplest  InputSameDT=on
      settings: InputPortMap=u0,u1
  For Each : ForEach  DisableCoverage=on
  Out1 : Outport  ConcatenationDimension=1  VectorParamsAs1DForOutWhenUnconnected=off
  wires:
  In1/1 -> 2-D Lookup Table/1
  2-D Lookup Table/1 -> Out1/1
  In2/1 -> 2-D Lookup Table/2

== system DriverInLoopSpeedgoat/Environment/Ground Height/3D Engine/Subsystem ==
  In1 : Inport
  Enable : EnablePort
  "Byte Unpacking " : slrealtimeutilitieslib/Byte Unpacking  MaskUnpackedDataTypes={'single'}  MaskUnpackedDataSizes={[4]}  MaskAlignment=1
      settings: SourceProductBaseCode=XP
  Rx Data : Outport
  wires:
  In1/1 -> "Byte Unpacking "/1
  "Byte Unpacking "/1 -> Rx Data/1  "Rx Data"

== system DriverInLoopSpeedgoat/Environment/Ground Height/3D Engine/While Iterator Subsystem ==
  Compare To Constant : simulink/Logic and Bit Operations/Compare To Constant  relop===  const=16  OutDataTypeStr=boolean
  Constant : Constant
  Subtract : Sum  Inputs=+-
  UDP Receive1 : slrealtimeiplib/UDP Receive  useHostTargetConn=off  ipAddress=target_ip  localPort=25002  rcvWidth=16  rcvFmAny=off  fmAddress=host_ip  sampleTime=-1
      settings: SourceProductBaseCode=XP
  While Iterator : WhileIterator  MaxIters=10  WhileBlockType=do-while  ShowIterationPort=on
  Data : Outport
  NumMsg : Outport  Port=2
  wires:
  UDP Receive1/2 -> Compare To Constant/1
  Compare To Constant/1 -> While Iterator/1
  While Iterator/1 -> Subtract/1
  Constant/1 -> Subtract/2
  Subtract/1 -> NumMsg/1
  UDP Receive1/1 -> Data/1

== system DriverInLoopSpeedgoat/External Driver Input/External Driver - Speedgoat/MapAndScaleAxes/conv to steering angle ==
  Steering Angle Filt : Inport
  Counts2Deg : Gain  Gain=(900)/65535
  Deg2Rad : Gain  Gain=2*pi/360
  SteerAngleBias : Constant  Value=450
  Sum : Sum  Inputs=|+-
  SteeringAngle : Outport  VectorParamsAs1DForOutWhenUnconnected=off
  wires:
  Sum/1 -> Deg2Rad/1  "steerAngleExternDeg"
  Steering Angle Filt/1 -> Counts2Deg/1  "steerAngleFiltCnts"
  Counts2Deg/1 -> Sum/1
  SteerAngleBias/1 -> Sum/2
  Deg2Rad/1 -> SteeringAngle/1  "steerAngleExternRad"

== matlab function DriverInLoopSpeedgoat/refgen ==
  data: w output; x input; omega input; des output; steer_cmd input; Fx input; Fy input; yyd output; fr output; par data_store_memory
function [w, des, yyd, fr] = refgen(x,omega,steer_cmd,Fx,Fy)
% x = [u, v, r]
% w = [delta, w1, w2, w3, w4]
% par = [str_ratio, m, Iz, L, lf, lr, Cy, Cx, trk_width, R_eff, g, Kus, Cd]'

global par;
p1 = par(4);
p2 = par(12)/par(11);
q1 = par(6);
q2 = -(par(5)*par(2))/(par(7)*par(4));
q = 2*(p1*q2-p2*q1);
delta = steer_cmd/par(1);
w = [delta; omega];

F_X1 = Fx(1)+Fx(2);         % F_Xf
F_X2 = Fx(3)+Fx(4);
F_Y1 = Fy(1)+Fy(2);
F_Y2 = Fy(3)+Fy(4);         % F_Yr
F_X = F_X1*cos(delta)-F_Y1*sin(delta)+F_X2;         % F_X total on veh
F_Y = F_X1*sin(delta)+F_Y1*cos(delta)+F_Y2;         % F_Y total on veh

% f1 = ax;
% f2 = ay;
f1 = 1/par(2)*(F_X-par(13)*x(1)^2)+x(2)*x(3);
f2 = 1/par(2)*F_Y-x(1)*x(3);
fr = 1/par(3)*(par(5)*(F_X1*sin(delta)+F_Y1*cos(delta))-par(6)*F_Y2);            % rdot without u,d
des1 = delta*(q1+q2*x(1)^2)/(p1+p2*x(1)^2);             % beta_des
des2 = x(1)*delta/(p1+p2*x(1)^2);                       % r_des
desdot1 = q*x(1)*f1*delta/(p1+p2*x(1)^2)^2;             % beta_des_dot
desdot2 = (p1-p2*x(1)^2)*f1*delta/(p1+p2*x(1)^2)^2;     % r_des_dot
des = [des1; des2; desdot1; desdot2];
e_beta = atan(x(2)/x(1))-des1;
e_r = x(3)-des2;
e_beta_dot = (x(1)*f2-x(2)*f1)/(x(1)^2+x(2)^2)-desdot1;
yyd = double([e_beta, e_r, e_beta_dot]');

end

== matlab function DriverInLoopSpeedgoat/ET-SMC ==
  data: x input; w input; des input; yyd input; f_r input; Mz output; mode input; simtime input
function Mz  = fcn(x, w, des, yyd, f_r, mode, simtime)
% xw = [u,u,r,delta,w1,w2,w3,w4]'
% yyd = [e_beta, e_r, e_beta_dot]'
% des = [beta, r, betadot, rdot]
% F_tyre = [xfl,-,-,xrr,yfl,-,-,yrr]'
% par = [str_ratio, m, Iz, L, lf, lr, Cyf, Cyr, trk_width, R_eff, g]'
% mode = 1 for ETC, 0 for Periodic

global event par;
Lh = 11.148;
Le = 193.547;
xi = -1.5;
gamma = 5;
eta = 7.5;
c = [xi; 1];
x = xw(1:3);
w = xw(4:8);
nu = 0.015;          % inverse slope

%% Ct-SMC
s = xi*yyd(1)+yyd(2);
sat_s = sign(s)*min(1,abs(s/nu));   % high slope saturation
if x(1)>=6.95 && abs(yyd(2))>=0.02
%     u_c = single(-par(3)*(f_r + xi*yyd(3)-des(3) + eta*sign(s)));
    u_c = single(-par(3)*(f_r + xi*yyd(3)-des(3) + eta*sat_s));
else
    u_c = single(0);
end

Mz = single(u_c);
%% ET-SMC
% event(1:11) --> [xk(3), wk(5), yk(2), uk(1), simtime]'
if mode == 1                                % ETC chosen
    xk = event(1:3);
    wk = event(4:8);
    uk = event(11);
    
    if uk~=0                                        % ESP active already
        if norm([x;w]-[xk;wk])>= gamma/(Le*norm(c))     % Update control action
            event(1:3) = x;
            event(4:8) = w;
            event(9:10) = yyd(1:2);
            event(11) = u_c;                                % Update control
            Mz = single(event(11));
            event(12) = simtime;                            
            event(13) = event(13)+1;                        % Increase event count
        elseif abs(yyd(2))<0.02 || x(1)<6.95           % ESP action not required anymore
            event(1:3) = x;
            event(4:8) = w;
            event(9:10) = [0,0]';                           % Errors = 0
            event(11) = 0;                                  % Control = 0
            Mz = single(event(11));
            event(12) = simtime;                            
            event(13) = event(13)+1;                        % Increase event count
        end
    elseif abs(yyd(2))>=0.02 && x(1)>=6.95          % inactive but ACTIVATE NOW
        event(1:3) = x;
        event(4:8) = w;
        event(9:10) = yyd(1:2);
        event(11) = u_c;                                % Update control
        Mz = single(event(11));
        event(12) = simtime;                            
        event(13) = event(13)+1;                        % Increase event count
    end
    
end
end
%%

== stateflow chart DriverInLoopSpeedgoat/Controllers/Transmission Controller/Chart ==
  state Automatic
    entry:
    Mode = 1;
    during:
    if (elapsed(sec) >=1)
    debounce=0;
    end
  state Manual
    entry:
    Mode = 0;
    during:
    if (elapsed(sec) >=1)
    debounce=0;
    end
  (default) -> Automatic
  Manual -> Automatic : [Toggle==1 && debounce==0] {debounce=1}
  Automatic -> Manual : [Toggle==1 && debounce==0] {debounce=1}
  data: Toggle input; Mode output; debounce local =0

== stateflow chart DriverInLoopSpeedgoat/Controllers/Transmission Controller/Automatic/TCM Shift Controller ==
  settings: sampleTime=0.01
  state GearCmd [parallel]
    settings: executionOrder=1
    state Neutral
      en:
      GearCmd = 0;
    state G1
      en:
      GearCmd = 1;
    state G2
      en:
      GearCmd = 2;
      du:
      [SpdThr] = calc(2,pedal,speed);
    state G3
      en:
      GearCmd = 3;
      du:
      [SpdThr] = calc(3,pedal,speed);
    state G5
      en:GearCmd=5;
      du:[SpdThr]=calc(5,pedal,speed);
    state G4
      en:
      GearCmd = 4;
      du:
      [SpdThr] = calc(4,pedal,speed);
    (default) -> G1
    Neutral -> G1 : [~Neutral]
    G1 -> G2 [order 1] : Up
    G2 -> G3 [order 1] : Up
    G1 -> Neutral [order 2] : [Neutral]
    G2 -> G1 [order 2] : Down
    G3 -> G2 [order 2] : Down
    G3 -> G4 [order 1] : Up
    G4 -> G3 [order 2] : Down
    G4 -> G5 [order 1] : Up
    G5 -> G4 : Down
  state SelectionState [parallel]
    du:[up_th]=calc_up(GearCmd,pedal);
    du:[down_th]=calc_down(GearCmd,pedal);
    settings: executionOrder=2
    state SteadyState
      en:
      clutchControl = 0;
    state preDownShifting
    state preUpShifting
    state UpShifting
      en:
      GearCmd = GearCmd + 0.5;
    state DownShifting
      en:
      GearCmd = GearCmd - 0.5;
    (default) -> SteadyState
    SteadyState -> (junction 62) [order 1] : [speed < down_th && ...
        | GearCmd >1]
    SteadyState -> (junction 128) [order 2] : [speed > up_th &&...
        | GearCmd <= 4 && ...
        | floor(GearCmd) == GearCmd]
    (junction 62) -> preDownShifting
    (junction 128) -> preUpShifting
    (junction 168) -> SteadyState
    (junction 23) -> SteadyState
    (junction 161) -> SteadyState
    preDownShifting -> (junction 168) [order 2] : [speed >= down_th]
    preUpShifting -> (junction 161) [order 2] : [speed <= up_th]
    preUpShifting -> UpShifting [order 1] : after(0.5,sec)
        | [speed>up_th]
    preDownShifting -> DownShifting [order 1] : after(0.5, sec)
        | [speed < down_th - 2]
    DownShifting -> (junction 23) : {GearCmd.Down;}
    UpShifting -> (junction 23) : {GearCmd.Up;}
  state up_th = calc_up(gear,pedal) [function]
  state down_th = calc_down(gear,pedal) [function]
  state SpdThr = calc(gear,pedal,speed) [function]
  data: gear function_input; pedal function_input; up_th function_output; gear function_input; pedal function_input; down_th function_output; gear function_input; pedal function_input; SpdThr function_output; speed function_input; GearCmd output int8; speed input; pedal input; clutchControl local double; SpdThr local double; Neutral input; up_th local double; down_th local double
  events: Up local EITHER_EDGE_EVENT; Down local EITHER_EDGE_EVENT
